simulink model "sim12a"  (R2015a)
settings: Solver=ode45  StartTime=0.0  StopTime=10.0  RelTol=1e-3
values from neighbouring files (symbols this model uses):
  b = 0    [lab2.m]
  yinicial = 1    [lab2.m]
  ypinicial = 0    [lab2.m]
settings Model: Creator=Pedro  LastModifiedBy=Pedro

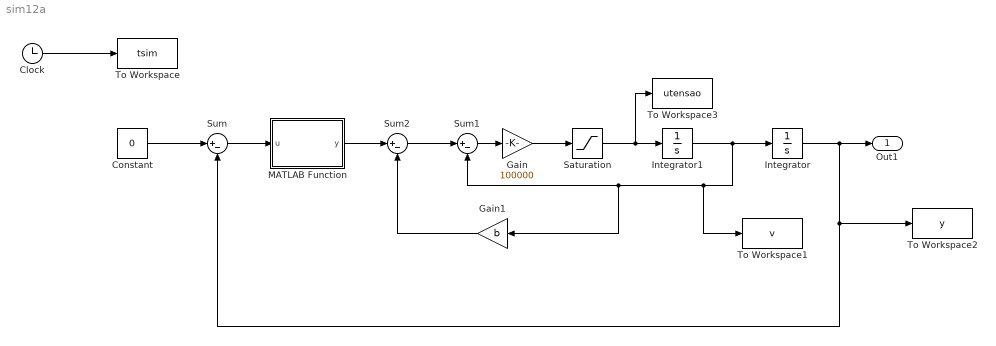
== system sim12a ==
  Clock : Clock
  Constant : Constant  Value=0
  Gain : Gain  Gain=100000
  Gain1 : Gain  Gain=b
  Integrator : Integrator  InitialCondition=yinicial
  Integrator1 : Integrator  InitialCondition=ypinicial
  MATLAB Function : MATLAB Function  TreatAsAtomicUnit=on
  Saturation : Saturate  UpperLimit=1  LowerLimit=-1
  Sum : Sum  Inputs=|+-
  Sum1 : Sum  Inputs=|+-
  Sum2 : Sum  Inputs=|+-
  To Workspace : ToWorkspace  VariableName=tsim  SampleTime=-1
  To Workspace1 : ToWorkspace  VariableName=v  SampleTime=-1
  To Workspace2 : ToWorkspace  VariableName=y  SampleTime=-1
  To Workspace3 : ToWorkspace  VariableName=utensao  SampleTime=-1
  Out1 : Outport
  wires:
  Sum1/1 -> Gain/1
  Gain/1 -> Saturation/1
  Saturation/1 -> To Workspace3/1, Integrator1/1
  Integrator1/1 -> To Workspace1/1, Gain1/1, Sum1/2, Integrator/1
  Constant/1 -> Sum/1
  Integrator/1 -> To Workspace2/1, Sum/2, Out1/1
  Clock/1 -> To Workspace/1
  Sum/1 -> MATLAB Function/1(u)
  Sum2/1 -> Sum1/1
  MATLAB Function/1(y) -> Sum2/1
  Gain1/1 -> Sum2/2

== matlab function sim12a/MATLAB Function ==
  data: u input; y output
function y = fcn(u)
%#codegen

y = sign(u)*sqrt(2*abs(u));
